simulink model "Incremental_Conductance"  (R2017b)
settings: Solver=VariableStepAuto  StartTime=0.0  StopTime=10.0  RelTol=1e-3
settings Model: Creator=SeanP  LastModifiedBy=SeanP

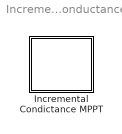
== system Incremental_Conductance ==
  Incremental Condictance MPPT : Stateflow chart  TreatAsAtomicUnit=on

== stateflow chart Incremental_Conductance/Incremental Condictance MPPT ==
  state SAMPLE_and_CALCULATE
    entry:
    deltaV = Vpv - Vprev;
    deltaI = Ipv - Iprev;
    Vguess = Vmpp;
  state INCREASE_VOLTAGE
    entry:
    Vguess = Vguess + Vincrement
  state DECREASE_VOLTAGE
    entry:
    Vguess = Vguess - Vincrement
  state INCREASE_VOLTAGE1
    entry:
    Vguess = Vguess + Vincrement
  state DECREASE_VOLTAGE1
    entry:
    Vguess = Vguess - Vincrement
  state Return
    entry:
    Vprev = Vpv;
    Iprev = Ipv;
    Vmpp = Vguess;
  (default) -> SAMPLE_and_CALCULATE
  (junction 44) -> SAMPLE_and_CALCULATE
  SAMPLE_and_CALCULATE -> (junction 52)
  (junction 52) -> (junction 5) [order 2] : [DeltaV == 0]
  (junction 52) -> (junction 4) [order 1]
  (junction 45) -> (junction 44)
  (junction 5) -> Return [order 3] : % At MPP
  (junction 4) -> Return [order 3] : [deltaV < -Vtol || deltaV > Vtol]
  (junction 5) -> DECREASE_VOLTAGE1 [order 2] : [deltaI > 0 ]
  (junction 4) -> INCREASE_VOLTAGE [order 1] : [deltaI/deltaV < -Ipv/Vpv]
  (junction 4) -> DECREASE_VOLTAGE [order 2] : [deltaI/deltaV > -Ipv/Vpv]
  (junction 5) -> INCREASE_VOLTAGE1 [order 1] : [deltaI < 0 ]
  INCREASE_VOLTAGE -> Return
  DECREASE_VOLTAGE -> Return
  INCREASE_VOLTAGE1 -> Return
  DECREASE_VOLTAGE1 -> Return
  Return -> (junction 45)
